simulink model "Model_control"  (R2023b)
settings: Solver=VariableStepAuto  StartTime=0.0  StopTime=10.0  RelTol=1e-3
values from neighbouring files (symbols this model uses):
  L = 0.000333    [Use_this_for_PI.m]
  R = 3.17    [Use_this_for_PI.m]
undefined symbols (not defined in the file or in its folder): J, Kd, kf, kt, N1, N2, N3, N4
settings Model: Creator=Aleks  LastModifiedBy=Aleks

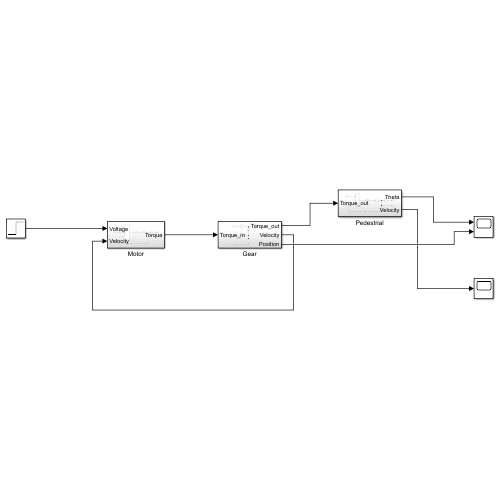
[thumbnail: Simulink's stored preview of the top-level diagram]
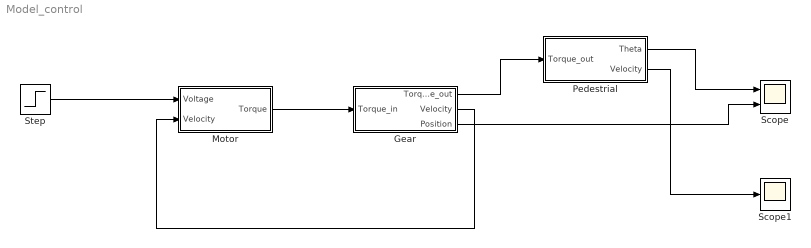
== system Model_control ==
  Gear : Subsystem
  Motor : Subsystem
  Pedestrial : Subsystem
  Scope : Scope  NumInputPorts=2
  Scope1 : Scope
  Step : Step  SampleTime=0
  wires:
  Gear/1(Torque_out) -> Pedestrial/1(Torque_out)
  Motor/1(Torque) -> Gear/1(Torque_in)
  Gear/2(Velocity) -> Motor/2(Velocity)
  Step/1 -> Motor/1(Voltage)
  Pedestrial/1(Theta) -> Scope/1
  Gear/3(Position) -> Scope/2
  Pedestrial/2(Velocity) -> Scope1/1

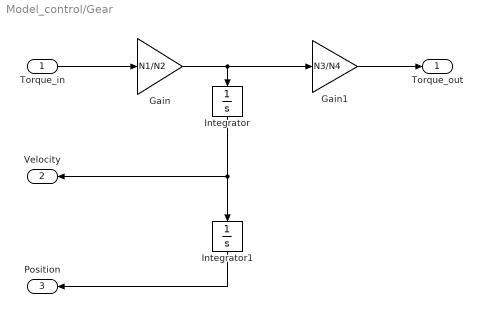
== system Model_control/Gear ==
  Torque_in : Inport
  Gain : Gain  Gain=N1/N2
  Gain1 : Gain  Gain=N3/N4
  Integrator : Integrator
  Integrator1 : Integrator
  Torque_out : Outport
  Velocity : Outport  Port=2
  Position : Outport  Port=3
  wires:
  Torque_in/1 -> Gain/1
  Gain/1 -> Gain1/1, Integrator/1
  Gain1/1 -> Torque_out/1
  Integrator/1 -> Integrator1/1, Velocity/1
  Integrator1/1 -> Position/1

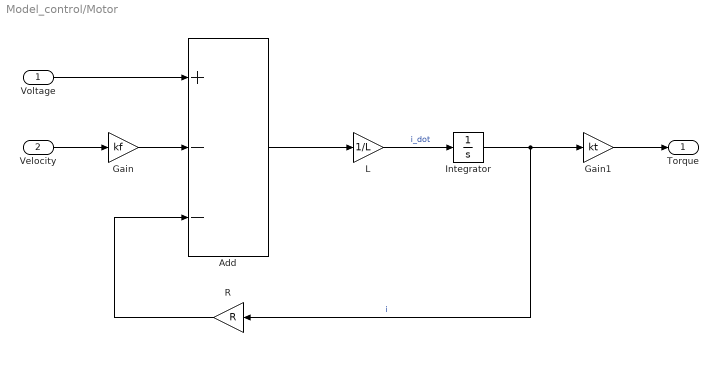
== system Model_control/Motor ==
  Voltage : Inport
  Velocity : Inport  Port=2
  Add : Sum  Inputs=+--
  Gain : Gain  Gain=kf
  Gain1 : Gain  Gain=kt
  Integrator : Integrator
  L : Gain  Gain=1/L
  R : Gain  Gain=R
  Torque : Outport
  wires:
  Gain1/1 -> Torque/1
  Gain/1 -> Add/2
  Integrator/1 -> Gain1/1, R/1  "i"
  Voltage/1 -> Add/1
  R/1 -> Add/3
  Velocity/1 -> Gain/1
  L/1 -> Integrator/1  "i_dot"
  Add/1 -> L/1

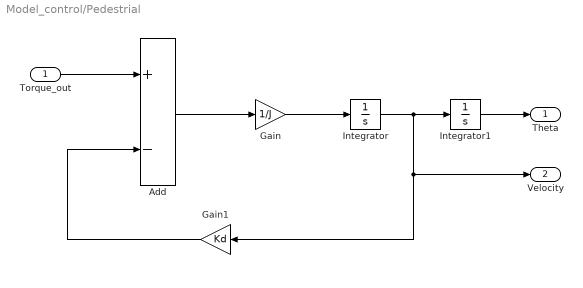
== system Model_control/Pedestrial ==
  Torque_out : Inport
  Add : Sum  Inputs=+-
  Gain : Gain  Gain=1/J
  Gain1 : Gain  Gain=Kd
  Integrator : Integrator
  Integrator1 : Integrator
  Theta : Outport
  Velocity : Outport  Port=2
  wires:
  Torque_out/1 -> Add/1
  Add/1 -> Gain/1
  Gain/1 -> Integrator/1
  Integrator/1 -> Integrator1/1, Velocity/1, Gain1/1
  Gain1/1 -> Add/2
  Integrator1/1 -> Theta/1
